simulink model "Final_Model"  (R2024a)
settings: Solver=VariableStepAuto  StartTime=0.0  StopTime=10.0  RelTol=1e-3
values from neighbouring files (symbols this model uses):
  G = 5    [K_mat.m]    (also in init.m)
  H = 1    [K_mat.m]    (also in init.m)
  K = -V/Z    [solveKMatrix_class.m]
  L = 20    [K_mat.m]    (also in init.m)
  M = 100    [K_mat.m]    (also in init.m)
  R = 3    [K_mat.m]    (also in control.m = 1; init.m)
  x_ref = [0.01, 0, 0.002]    [control.m]
settings Model: Creator=casager  LastModifiedBy=casager

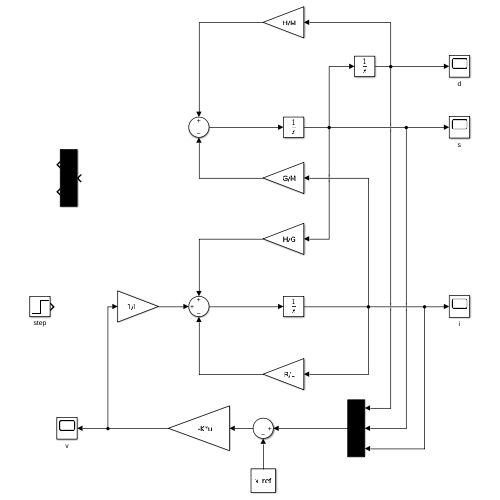
[thumbnail: Simulink's stored preview of the top-level diagram]
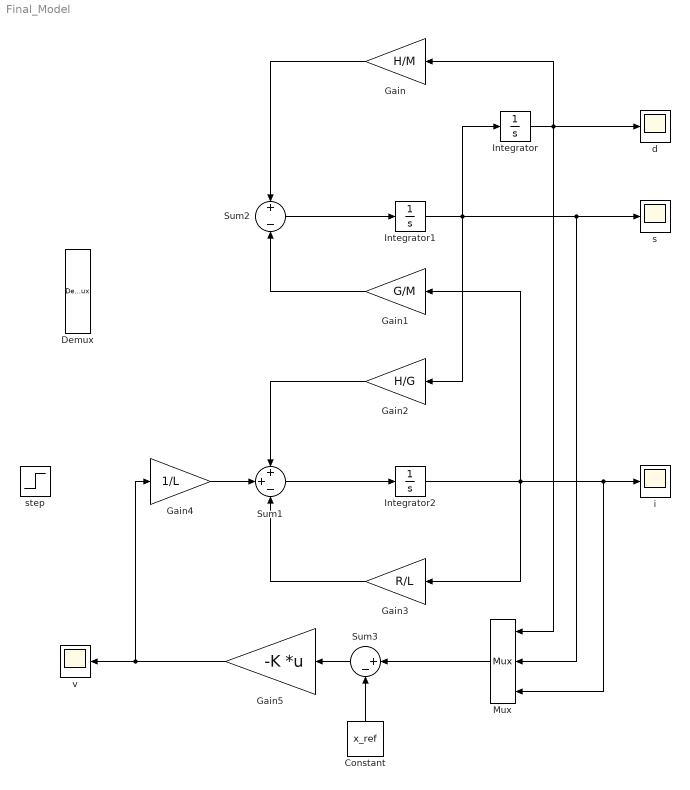
== system Final_Model ==
  Constant : Constant  Value=x_ref
  Demux : Demux  Outputs=2
  Gain : Gain  Gain=H/M
  Gain1 : Gain  Gain=G/M
  Gain2 : Gain  Gain=H/G
  Gain3 : Gain  Gain=R/L
  Gain4 : Gain  Gain=1/L
  Gain5 : Gain  Gain=-K  Multiplication=Matrix(K*u)
  Integrator : Integrator  InitialCondition=.02
  Integrator1 : Integrator
  Integrator2 : Integrator
  Mux : Mux  Inputs=3
  Sum1 : Sum  Inputs=++-
  Sum2 : Sum  Inputs=+-
  Sum3 : Sum  Inputs=|+-
  d : Scope
  i : Scope
  s : Scope
  step : Step  After=100  SampleTime=0
  v : Scope
  wires:
  Gain4/1 -> Sum1/2
  Integrator1/1 -> Integrator/1, Gain2/1, Mux/2, s/1
  Integrator2/1 -> Gain1/1, Mux/3, i/1, Gain3/1
  Gain3/1 -> Sum1/3
  Sum1/1 -> Integrator2/1
  Gain/1 -> Sum2/1
  Gain1/1 -> Sum2/2
  Gain2/1 -> Sum1/1
  Sum2/1 -> Integrator1/1
  Integrator/1 -> Mux/1, Gain/1, d/1
  Gain5/1 -> v/1, Gain4/1
  Mux/1 -> Sum3/1
  Sum3/1 -> Gain5/1
  Constant/1 -> Sum3/2
